simulink model "klasyk"  (Simulink 7.9)
settings: Solver=ode45  StartTime=0.0  StopTime=50  RelTol=1e-3
settings Model: Creator=student  LastModifiedBy=student

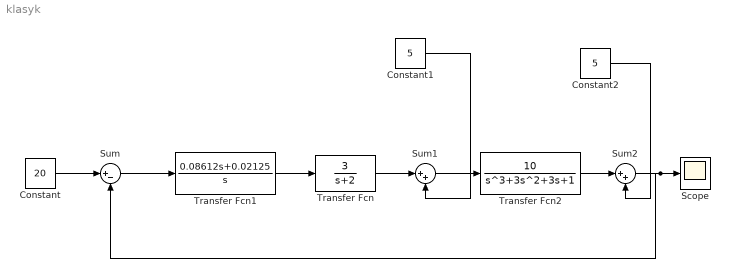
== system klasyk ==
  Constant : Constant  Value=20
  Constant1 : Constant  Value=5
  Constant2 : Constant  Value=5
  Scope : Scope
  Sum : Sum  Inputs=|+-
  Sum1 : Sum  Inputs=|++
  Sum2 : Sum  Inputs=|++
  Transfer Fcn : TransferFcn  Numerator=[3]  Denominator=[1 2]
  Transfer Fcn1 : TransferFcn  Numerator=[0.08612 0.02125]  Denominator=[1 0]
  Transfer Fcn2 : TransferFcn  Numerator=[10]  Denominator=[1 3 3 1]
  wires:
  Sum/1 -> Transfer Fcn1/1
  Transfer Fcn1/1 -> Transfer Fcn/1
  Transfer Fcn2/1 -> Sum2/1
  Constant2/1 -> Sum2/2
  Sum2/1 -> Scope/1, Sum/2
  Transfer Fcn/1 -> Sum1/1
  Constant1/1 -> Sum1/2
  Sum1/1 -> Transfer Fcn2/1
  Constant/1 -> Sum/1
